simulink library "MagLevTbx_BaseLib"  (R2025b)
settings: Solver=VariableStepAuto  StartTime=0.0  StopTime=10.0  RelTol=1e-3
undefined symbols (not defined in the file or in its folder): DiscIntNeverNeededParam
libraries: simulink x1
settings Model: Creator=riccardo  LastModifiedBy=riccardo
settings SolverCC: AlgebraicLoopSolver=TrustRegion
settings DataIOCC: ReturnWorkspaceOutputs=off
settings DebuggingCC: UnconnectedInputMsg=warning  UnconnectedOutputMsg=warning  UnconnectedLineMsg=warning  ArithmeticOperatorsInVariantConditions=warning
settings ModelReferenceCC: EnableRefExpFcnMdlSchedulingChecks=on
settings SFSimCC: SimUseLocalCustomCode=off  CustomCodeUndefinedFunction=UseInterfaceOnly
settings RTWCC: RTWUseLocalCustomCode=off  GPUComputeCapability=3.5  DLArmComputeVersion=19.05

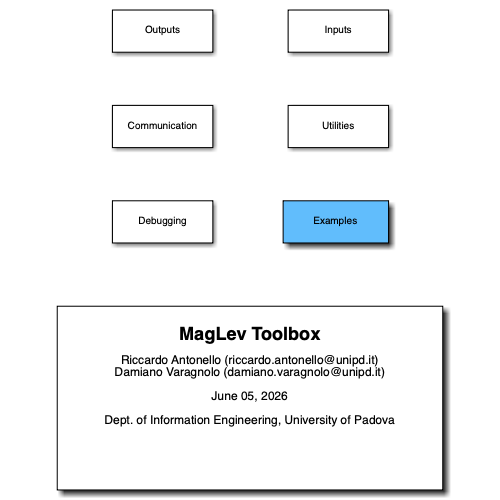
[thumbnail: Simulink's stored preview of the top-level diagram]
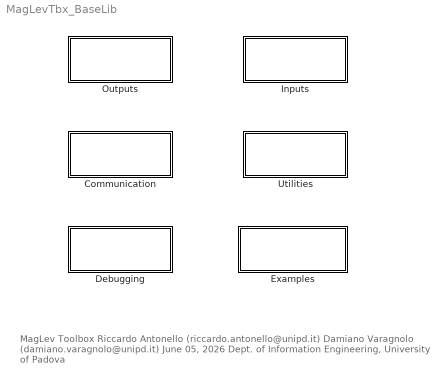
== system MagLevTbx_BaseLib ==
  note: MagLev Toolbox
      |
      | Riccardo Antonello (riccardo.antonello@unipd.it)
      | Damiano Varagnolo (damiano.varagnolo@unipd.it)
      |
      | June 05, 2026
      |
      | Dept. of Information Engineering, University of Padova
  Communication : Subsystem
      mask Display: disp(get_param(gcb,'name'))
  Debugging : Subsystem
      mask Display: disp(get_param(gcb,'name'))
  Examples : Subsystem  mask{ShowInLibBrowser=on}
      settings: OpenFcn=|
      | %  get toolbox root dir
      | info = MagLevTbx_Info();
      | 
      | %  path to demos
      | sldemopath = fullfile( info.rootDir, ...
      | 'Examples', ...
      | 'MagLevTbx_Demos' );
      | 
      | %  open demo
      | open_system( sldemopath, 'force' );
      | 
      | %  clear temp vars
      | clear info sldemopath;
      mask Display: disp(get_param(gcb,'name'))
  Inputs : Subsystem
      mask Display: disp(get_param(gcb,'name'))
  Outputs : Subsystem
      mask Display: disp(get_param(gcb,'name'))
  Utilities : Subsystem
      mask Display: disp(get_param(gcb,'name'))

== system MagLevTbx_BaseLib/Communication ==
  USB Serial Packet Receive : Subsystem  mask(USB Serial Packet Receive){outputMode=HOLD Outputs, showStatusPort=on, packetSpec={'uint8', 'uint16', 'double'}, cobsEncoded=on, nullTerminated=on, sampleTime=-1, showEnablePort=off}
      mask prompts: outputMode "In case of missing packet:"; showStatusPort "Show status port"; packetSpec "Packet Specifier ( e.g. {'2*uint8', '3*single'} ):"; cobsEncoded "COBS Encoded"; nullTerminated "Null Terminated"; sampleTime "Sample time (-1 for inherited):"; showEnablePort "Show enable port"
      mask help:
      | Receive data packet from the USB serial port.
      |
      | The Status Port is set to a nonzero value when a new packet has been correctly received, and new data is available at the output ports.
      mask init:
      | cobsEncoded = logical(cobsEncoded);
      | nullTerminated = logical(nullTerminated);
      | showStatusPort = logical(showStatusPort);
      | 
      | %   init block
      | MagLevTbx_UsbSerialPacketReceive_MaskInit(gcb, packetSpec, showStatusPort, showEnablePort);
      mask Help:
      | Riccardo Antonello (riccardo.antonello@unipd.it)
      | 
      | February 18, 2026
      | 
      | Dept. of Information Engineering, University of Padova
      mask TypeOptions outputMode: HOLD Outputs | RESET Outputs
      mask Callback sampleTime: MagLevTbx_UsbSerialPacketReceive_MaskCbFcn_SampleTime();
      mask DialogControl Container3 Prompt: Communication link
      mask DialogControl Container4 Prompt: Packet definition
  USB Serial Packet Send : Subsystem  mask(USB Serial Packet Send){waitDTR=on, packetSpec={'uint8', 'int16', 'single'}, cobsEncoded=on, nullTerminated=on, sampleTime=-1, showEnablePort=off}
      mask prompts: waitDTR "Wait for DTR signal"; packetSpec "Packet Specifier ( e.g. {'2*uint8', '3*single'} ):"; cobsEncoded "COBS Encoded"; nullTerminated "Null Terminated"; sampleTime "Sample time (-1 for inherited):"; showEnablePort "Show enable port"
      mask help: Send data packet using the USB serial port.
      mask init:
      | %   convert enable checkbox parameters to logical
      | cobsEncoded = logical(cobsEncoded);
      | nullTerminated = logical(nullTerminated);
      | waitDTR = logical(waitDTR);
      | 
      | %   init block
      | MagLevTbx_UsbSerialPacketSend_MaskInit(gcb, packetSpec, showEnablePort);
      mask Help:
      | Riccardo Antonello (riccardo.antonello@unipd.it)
      | 
      | February 18, 2026
      | 
      | Dept. of Information Engineering, University of Padova
      mask Callback sampleTime: MagLevTbx_UsbSerialPacketSend_MaskCbFcn_SampleTime();
      mask DialogControl Container4 Prompt: Communication link
      mask DialogControl Container3 Prompt: Packet definition

== system MagLevTbx_BaseLib/Debugging ==
  Execution Pause : Subsystem  mask(Execution Pause){pauseTime=10}
      mask prompts: pauseTime "Execution pause [us]:"
      mask help: Insert an execution pause of specified microseconds in the model step routine.
      mask Help:
      | Riccardo Antonello (riccardo.antonello@unipd.it)
      | 
      | June 05, 2026
      | 
      | Dept. of Information Engineering, University of Padova
  Execution Time : Subsystem  mask(Execution Time){digitalPinEnable=off, digitalPin=0}
      mask prompts: digitalPinEnable "Enable digital pin"; digitalPin "Pin number:"
      mask help:
      | Measure the execution time of a model (or atomic block) step routine.
      |
      | The measurement resolution is of 1 microseconds.
      |
      | A digital output pin can be optionally enabled to monitor the execution of the step routine; the pin is set to HIGH during the execution of the step routine, and reset otherwise.
      |
      | To monitor the execution time of a subsystem, place the block within the subsystem, and force the subsystem to be an atomic-block.
      mask Help:
      | Riccardo Antonello (riccardo.antonello@unipd.it)
      | 
      | June 05, 2026
      | 
      | Dept. of Information Engineering, University of Padova
      mask Callback digitalPinEnable: MagLevTbx_ExecTime_MaskCbFcn_digitalPinEnable;
      mask Callback digitalPin: MagLevTbx_ExecTime_MaskCbFcn_digitalPin()

== system MagLevTbx_BaseLib/Examples ==

== system MagLevTbx_BaseLib/Inputs ==
  Current Sensor : Subsystem  mask(Current Sensor (Texas Instruments INA214A)){sensorId=+X, sampleTime=-1, showEnablePort=off}
      mask prompts: sensorId "Current sensor:"; sampleTime "Sample time (-1 for inherited):"; showEnablePort "Show enable port"
      mask help: Get current measurement (in [A]) from the selected current sensor.
      mask init:
      | MagLevTbx_CurrSens_MaskInit(gcb, showEnablePort);
      mask Help:
      | Riccardo Antonello (riccardo.antonello@unipd.it)
      | 
      | February 17, 2026
      | 
      | Dept. of Information Engineering, University of Padova
      mask Callback sampleTime: MagLevTbx_CurrSens_MaskCbFcn_SampleTime();
  Magnetic Sensor : Subsystem  mask(Magnetic Sensor (Infineon TLV493D)){sensorId=Sensor 7, sampleTime=-1, showEnablePort=off}
      mask prompts: sensorId "Magnetic Sensor:"; sampleTime "Sample time (-1 for inherited):"; showEnablePort "Show enable port"
      mask help: Get the 3D magnetic flux density 𝐵 in [𝑚𝑇] along the three sensor axes directions (𝑥,𝑦,𝑧).
      mask init:
      | %   select block variant according to hardware (PCB) version
      | blk = gcb;
      | vss = [blk '/MagSens'];
      | 
      | m = Simulink.Mask.get(gcb);
      | pSensorId = m.getParameter('sensorId');
      | 
      | group = "MagLevTbx";
      | pref  = "HwVersion";
      | 
      | if ispref(group, pref)
      |     hwVer = getpref(group, pref);
      |     switch hwVer 
      |         case '4.0'
      |             set_param(vss, 'LabelModeActiveChoice', '4.0');
      |             pSensorId.Visible = 'on';
      |         case '4.3'
      |             set_param(vss, 'LabelModeActiveChoice', '4.3');
      |             pSensorId.Visible = 'off';
      |         otherwise
      |             error('Unsupported PCB version: %s', hwVer);
      |     end
      | else
      |     hwVer = 0;
      |     disp('ciao')
      |     error('MagLevTbx:PCBVersionNotConfigured', ...
      |         'MagLev PCB version not configured. Please run MagLevTbx_HwConfig() to set the hardware version.');
      | end
      | 
      | %   add/remove enable block
      | MagLevTbx_MagSens_MaskInit(gcb, showEnablePort);
      mask Help:
      | Riccardo Antonello (riccardo.antonello@unipd.it)
      | 
      | February 17, 2026
      | 
      | Dept. of Information Engineering, University of Padova
      mask Callback sampleTime: MagLevTbx_MagSens_MaskCbFcn_SampleTime();

== system MagLevTbx_BaseLib/Outputs ==
  Current Driver : Subsystem  mask(Current Driver (Allegro A4950)){driverId=+X, sampleTime=-1, showEnablePort=off}
      mask prompts: driverId "Current driver:"; sampleTime "Sample time (-1 for inherited):"; showEnablePort "Show enable port"
      mask help:
      | Set the PWM duty cycle of the selected current driver.
      |
      | A valid PWM duty cycle is a int16 in the range [-255, +255].
      mask init:
      | MagLevTbx_CurrDrv_MaskInit(gcb, showEnablePort);
      mask Help:
      | Riccardo Antonello (riccardo.antonello@unipd.it)
      | 
      | February 17, 2026
      | 
      | Dept. of Information Engineering, University of Padova
      mask Callback sampleTime: MagLevTbx_CurrDrv_MaskCbFcn_SampleTime();
  User LED : Subsystem  mask(User LED){sampleTime=-1, showEnablePort=off}
      mask prompts: sampleTime "Sample time (-1 for inherited):"; showEnablePort "Show enable port"
      mask help: Set the state of the User LED.
      mask init:
      | MagLevTbx_UserLED_MaskInit(gcb, showEnablePort);
      mask Help:
      | Riccardo Antonello (riccardo.antonello@unipd.it)
      | 
      | February 26, 2026
      | 
      | Dept. of Information Engineering, University of Padova
      mask Callback sampleTime: MagLevTbx_UserLED_MaskCbFcn_SampleTime();

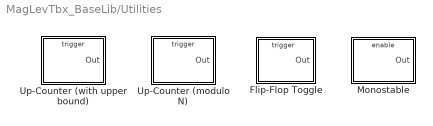
== system MagLevTbx_BaseLib/Utilities ==
  Flip-Flop Toggle : Subsystem  mask{y0_sel=LOW}
      mask prompts: y0_sel "Initial output"
      mask help:
      | Riccardo Antonello (riccardo.antonello@unipd.it)
      |
      | May 08, 2017
      |
      | Dept. of Information Engineering, University of Padova
      mask init:
      | if y0_sel == 1, 
      |     y0 = 0;
      |     s = 1;
      | else
      |     y0 = 1;
      |     s = 0;
      | end;
      mask TypeOptions y0_sel: LOW | HIGH
      mask DialogControl DescTextVar Prompt: Toggle output at each rising edge of the enable input
  Monostable : Subsystem  mask{Tp=1}
      mask prompts: Tp "Pulse duration [s]"
  Up-Counter (modulo N) : Subsystem  mask{N=10, C0=0}
      mask prompts: N "Counter modulo"; C0 "Counter init value"
      mask help:
      | Riccardo Antonello (riccardo.antonello@unipd.it)
      |
      | May 08, 2017
      |
      | Dept. of Information Engineering, University of Padova
      mask init:
      | if C0 < 0 || C0 > N, 
      |     C0 = 0;
      | end;
      mask DialogControl DescTextVar Prompt: Up-counter modulo N
  Up-Counter (with upper bound) : Subsystem  mask{CMAX=10, C0=0}
      mask prompts: CMAX "Counter upper bound"; C0 "Counter init value"
      mask help:
      | Riccardo Antonello (riccardo.antonello@unipd.it)
      |
      | May 08, 2017
      |
      | Dept. of Information Engineering, University of Padova
      mask init:
      | if CMAX < C0,
      |     CMAX = C0;
      | end;
      mask DialogControl DescTextVar Prompt: Up-counter with count upper bound

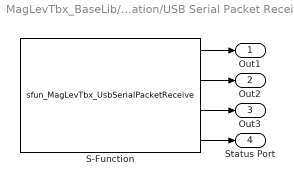
== system MagLevTbx_BaseLib/Communication/USB Serial Packet Receive ==
  S-Function : S-Function  FunctionName=sfun_MagLevTbx_UsbSerialPacketReceive  Parameters=packetSpec, cobsEncoded, nullTerminated, showStatusPort, outputMode, sampleTime  SFunctionDeploymentMode=off  EnableBusSupport=off
  Out1 : Outport
  Out2 : Outport  Port=2
  Out3 : Outport  Port=3
  Status Port : Outport  Port=4
  wires:
  S-Function/1 -> Out1/1
  S-Function/2 -> Out2/1
  S-Function/3 -> Out3/1
  S-Function/4 -> Status Port/1

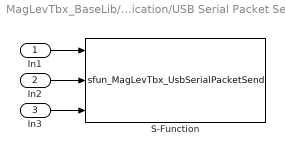
== system MagLevTbx_BaseLib/Communication/USB Serial Packet Send ==
  In1 : Inport
  In2 : Inport  Port=2
  In3 : Inport  Port=3
  S-Function : S-Function  FunctionName=sfun_MagLevTbx_UsbSerialPacketSend  Parameters=packetSpec, cobsEncoded, nullTerminated, waitDTR, sampleTime  SFunctionDeploymentMode=off  EnableBusSupport=off
  wires:
  In1/1 -> S-Function/1
  In2/1 -> S-Function/2
  In3/1 -> S-Function/3

== system MagLevTbx_BaseLib/Debugging/Execution Pause ==
  S-Function : S-Function  FunctionName=sfun_MagLevTbx_ExecPause  Parameters=pauseTime  SFunctionDeploymentMode=off  EnableBusSupport=off

== system MagLevTbx_BaseLib/Debugging/Execution Time ==
  S-Function : S-Function  FunctionName=sfun_MagLevTbx_ExecTime  Parameters=logical(digitalPinEnable), digitalPin  SFunctionDeploymentMode=off  EnableBusSupport=off
  Exec time [us] : Outport  VectorParamsAs1DForOutWhenUnconnected=off
  wires:
  S-Function/1 -> Exec time [us]/1

== system MagLevTbx_BaseLib/Inputs/Current Sensor ==
  S-Function : S-Function  FunctionName=sfun_MagLevTbx_CurrSens  Parameters=sensorId, sampleTime  SFunctionDeploymentMode=off  EnableBusSupport=off
  Current [A] : Outport
  wires:
  S-Function/1 -> Current [A]/1

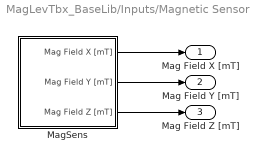
== system MagLevTbx_BaseLib/Inputs/Magnetic Sensor ==
  MagSens : Subsystem  Variant=on  VariantControlMode=label  LabelModeActiveChoice=4.0
  Mag Field X [mT] : Outport
  Mag Field Y [mT] : Outport  Port=2
  Mag Field Z [mT] : Outport  Port=3
  wires:
  MagSens/1(Mag Field X [mT]) -> Mag Field X [mT]/1
  MagSens/2(Mag Field Y [mT]) -> Mag Field Y [mT]/1
  MagSens/3(Mag Field Z [mT]) -> Mag Field Z [mT]/1

== system MagLevTbx_BaseLib/Outputs/Current Driver ==
  duty : Inport
  S-Function : S-Function  FunctionName=sfun_MagLevTbx_CurrDrv  Parameters=driverId, sampleTime  SFunctionDeploymentMode=off  EnableBusSupport=off
  wires:
  duty/1 -> S-Function/1

== system MagLevTbx_BaseLib/Outputs/User LED ==
  LED State : Inport
  S-Function : S-Function  FunctionName=sfun_MagLevTbx_UserLED  Parameters=sampleTime  SFunctionDeploymentMode=off  EnableBusSupport=off
  wires:
  LED State/1 -> S-Function/1

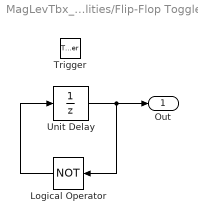
== system MagLevTbx_BaseLib/Utilities/Flip-Flop Toggle ==
  Trigger : TriggerPort  VariantControl=Variant  PortDimensions=1
  Logical Operator : Logic  Operator=NOT  AllPortsSameDT=off  OutDataTypeStr=boolean
  Unit Delay : UnitDelay  InitialCondition=s  SampleTime=-1  HasFrameUpgradeWarning=on
  Out : Outport  InitialOutput=y0  VectorParamsAs1DForOutWhenUnconnected=off
  wires:
  Logical Operator/1 -> Unit Delay/1
  Unit Delay/1 -> Out/1, Logical Operator/1

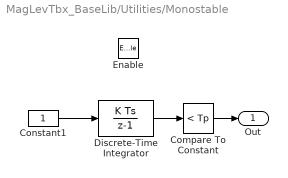
== system MagLevTbx_BaseLib/Utilities/Monostable ==
  Enable : EnablePort  StatesWhenEnabling=reset
  Compare To Constant : simulink/Logic and Bit Operations/Compare To Constant  relop=<  const=Tp  OutDataTypeStr=boolean
  Constant1 : Constant
  Discrete-Time Integrator : DiscreteIntegrator  SampleTime=-1  LimitOutput=on  UpperSaturationLimit=Tp  LowerSaturationLimit=0  ICPrevOutput=DiscIntNeverNeededParam  ICPrevScaledInput=DiscIntNeverNeededParam
  Out : Outport  VectorParamsAs1DForOutWhenUnconnected=off
  wires:
  Compare To Constant/1 -> Out/1
  Constant1/1 -> Discrete-Time Integrator/1
  Discrete-Time Integrator/1 -> Compare To Constant/1

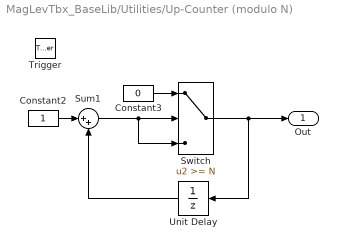
== system MagLevTbx_BaseLib/Utilities/Up-Counter (modulo N) ==
  Trigger : TriggerPort  VariantControl=Variant  PortDimensions=1
  Constant2 : Constant
  Constant3 : Constant  Value=0
  Sum1 : Sum  Inputs=|++
  Switch : Switch  Threshold=N  SaturateOnIntegerOverflow=off  InputSameDT=off
  Unit Delay : UnitDelay  InitialCondition=C0  SampleTime=-1  HasFrameUpgradeWarning=on
  Out : Outport  OutputWhenDisabled=reset  InitialOutput=C0  VectorParamsAs1DForOutWhenUnconnected=off
  wires:
  Switch/1 -> Out/1, Unit Delay/1
  Unit Delay/1 -> Sum1/2
  Sum1/1 -> Switch/2, Switch/3
  Constant2/1 -> Sum1/1
  Constant3/1 -> Switch/1

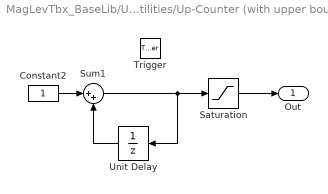
== system MagLevTbx_BaseLib/Utilities/Up-Counter (with upper bound) ==
  Trigger : TriggerPort  VariantControl=Variant  PortDimensions=1
  Constant2 : Constant
  Saturation : Saturate  UpperLimit=CMAX  LowerLimit=C0
  Sum1 : Sum  Inputs=|++
  Unit Delay : UnitDelay  InitialCondition=C0  SampleTime=-1  HasFrameUpgradeWarning=on
  Out : Outport  InitialOutput=C0  VectorParamsAs1DForOutWhenUnconnected=off
  wires:
  Sum1/1 -> Saturation/1, Unit Delay/1
  Unit Delay/1 -> Sum1/2
  Constant2/1 -> Sum1/1
  Saturation/1 -> Out/1

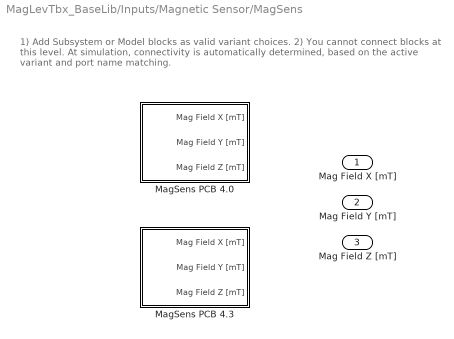
== system MagLevTbx_BaseLib/Inputs/Magnetic Sensor/MagSens ==
  note: 1) Add Subsystem or Model blocks as valid variant choices.
      | 2) You cannot connect blocks at this level. At simulation, connectivity is automatically
      | determined, based on the active variant and port name matching.
  MagSens PCB 4.0 : Subsystem  VariantControl=4.0
  MagSens PCB 4.3 : Subsystem  VariantControl=4.3
  Mag Field X [mT] : Outport
  Mag Field Y [mT] : Outport  Port=2
  Mag Field Z [mT] : Outport  Port=3

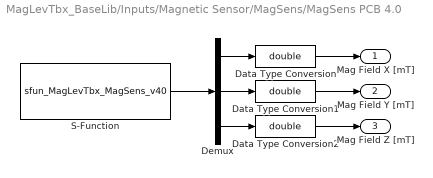
== system MagLevTbx_BaseLib/Inputs/Magnetic Sensor/MagSens/MagSens PCB 4.0 ==
  Data Type Conversion : DataTypeConversion  OutDataTypeStr=double  SaturateOnIntegerOverflow=off  RndMeth=Floor
  Data Type Conversion1 : DataTypeConversion  OutDataTypeStr=double  SaturateOnIntegerOverflow=off  RndMeth=Floor
  Data Type Conversion2 : DataTypeConversion  OutDataTypeStr=double  SaturateOnIntegerOverflow=off  RndMeth=Floor
  Demux : Demux  Outputs=3
  S-Function : S-Function  FunctionName=sfun_MagLevTbx_MagSens_v40  Parameters=sensorId, sampleTime  SFunctionDeploymentMode=off  EnableBusSupport=off
  Mag Field X [mT] : Outport
  Mag Field Y [mT] : Outport  Port=2
  Mag Field Z [mT] : Outport  Port=3
  wires:
  Data Type Conversion1/1 -> Mag Field Y [mT]/1
  Demux/2 -> Data Type Conversion1/1
  Demux/3 -> Data Type Conversion2/1
  Data Type Conversion/1 -> Mag Field X [mT]/1
  S-Function/1 -> Demux/1
  Demux/1 -> Data Type Conversion/1
  Data Type Conversion2/1 -> Mag Field Z [mT]/1

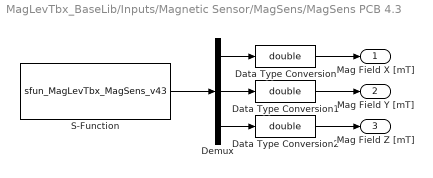
== system MagLevTbx_BaseLib/Inputs/Magnetic Sensor/MagSens/MagSens PCB 4.3 ==
  Data Type Conversion : DataTypeConversion  OutDataTypeStr=double  SaturateOnIntegerOverflow=off  RndMeth=Floor
  Data Type Conversion1 : DataTypeConversion  OutDataTypeStr=double  SaturateOnIntegerOverflow=off  RndMeth=Floor
  Data Type Conversion2 : DataTypeConversion  OutDataTypeStr=double  SaturateOnIntegerOverflow=off  RndMeth=Floor
  Demux : Demux  Outputs=3
  S-Function : S-Function  FunctionName=sfun_MagLevTbx_MagSens_v43  Parameters=sampleTime  SFunctionDeploymentMode=off  EnableBusSupport=off
  Mag Field X [mT] : Outport
  Mag Field Y [mT] : Outport  Port=2
  Mag Field Z [mT] : Outport  Port=3
  wires:
  Data Type Conversion2/1 -> Mag Field Z [mT]/1
  Demux/1 -> Data Type Conversion/1
  S-Function/1 -> Demux/1
  Data Type Conversion/1 -> Mag Field X [mT]/1
  Demux/3 -> Data Type Conversion2/1
  Demux/2 -> Data Type Conversion1/1
  Data Type Conversion1/1 -> Mag Field Y [mT]/1
